simulink model "model_6dof"  (R2021b)
settings: Solver=ode4  StartTime=0  StopTime=stopt  FixedStep=ts  RelTol=1e-3
values from neighbouring files (symbols this model uses):
  d = 0.265    [totalfm.m]
  q = U(2)    [totalfm.m]
  r = U(3)    [totalfm.m]
  rail_len = U(4)    [stage_func.m]
undefined symbols (not defined in the file or in its folder): afa, alpha, atkinter, beta, caoff1000, caoff10000, caoff5000, caon1000, caon10000, caon5000, cl_phi1000, cl_phi10000, cl_phi5000, cldp1000, cldp10000, cldp5000, clp10000, clp5000, clpc_1000, clpt_1000, cma_1000, cmad_1000, cmdq10000, cmdq5000, cmq1000, cmq10000, cmq5000, cn1000, cn10000, cn5000, cna_1000, cndq1000, cnq1000, cnq10000, cnq5000, damp, ex0, ey0, ez0, HDBK, K1, K2, K3, KP, MIL, Minter, p0, pitch_control_on, q0, r0, roll_control_on, Severe, SIM_CASE, tou, tou1, tou2, ts, turb_on, u0, v0 ... (+14)
libraries: simulink x15, simulink_extras x5, aerolibasang x2, dspmathops x1, aerolibatmos2 x1, aerolibconvert2 x1, aerolibwind2 x1, mspsensorlib x1, sensorinslib x1, sharedtransform x1, vrlib x1
settings Model: Creator=a0972  LastModifiedBy=310611102
settings DataIOCC: SaveFormat=StructureWithTime
settings OptimizationCC: BlockReduction=off  BufferReuse=off
settings DebuggingCC: AlgebraicLoopMsg=none  UnconnectedInputMsg=none  UnconnectedOutputMsg=none  UnconnectedLineMsg=none

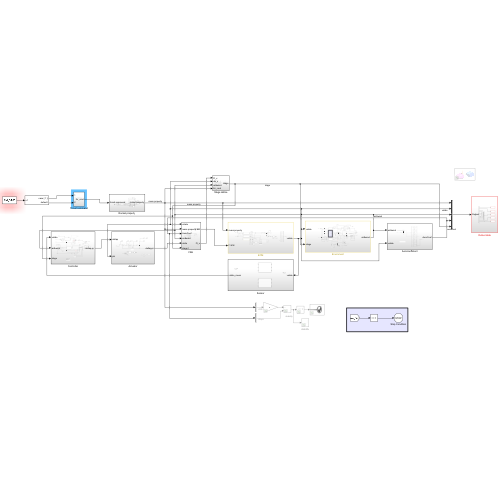
[thumbnail: Simulink's stored preview of the top-level diagram]
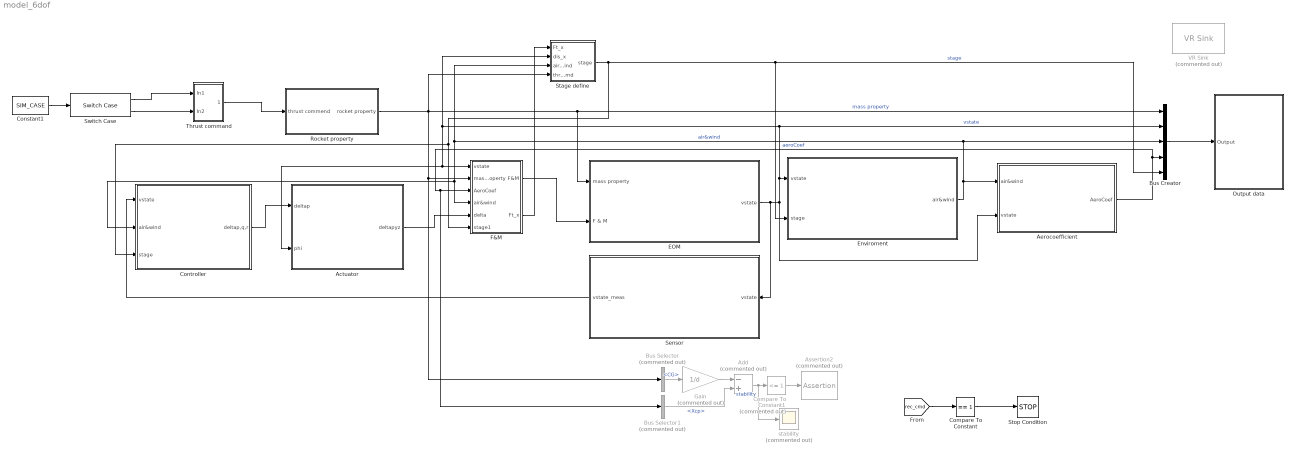
== system model_6dof ==
  Actuator : Subsystem
  Add : Sum  Commented=on  Inputs=-+
  Aerocoefficient : Subsystem
  Assertion2 : Assertion  Commented=on  AssertionFailFcn=error('unstable')
  Bus Creator : BusCreator  Inputs=5
  Bus Selector : BusSelector  Commented=on  OutputSignals=CG
  Bus Selector1 : BusSelector  Commented=on  OutputSignals=Xcp
  Compare To Constant : simulink/Logic and Bit Operations/Compare To Constant  relop===  const=1  OutDataTypeStr=boolean
  Compare To Constant1 : simulink/Logic and Bit Operations/Compare To Constant  Commented=on  relop=<=  const=1  OutDataTypeStr=boolean
  Constant1 : Constant  Value=SIM_CASE
  Controller : Subsystem
  EOM : Subsystem
  Enviroment : Subsystem
  F&M : Subsystem
  Gain : Gain  Commented=on  Gain=1/d
  Output data : Subsystem
  Rocket property : Subsystem
  Sensor : Subsystem
  Stage define : Subsystem
  Stop Condition : Stop
  Switch Case : SwitchCase
  Thrust command : Subsystem
  VR Sink : vrlib/VR Sink  Commented=on  InstantiateOnLoad=on  SampleTime=ts  ViewEnable=on  RemoteChange=off  RemoteView=off  AutoView=off  VideoDimensions=[]  AllowVariableSize=off
  stability : Scope  Commented=on
  wires:
  Controller/1(deltap,q,r) -> Actuator/1(deltap)
  Bus Creator/1 -> Output data/1(Output)
  EOM/1(vstate) -> Sensor/1(vstate), Bus Creator/2, F&M/1(vstate), Actuator/2(phi), Stage define/2(dis_x), Enviroment/1(vstate), Aerocoefficient/2(vstate)  "vstate"
  Rocket property/1(rocket property) -> Bus Selector/1, F&M/2(mass property), Stage define/4(thr_cmd), EOM/1(mass property), Bus Creator/1  "mass property"
  Aerocoefficient/1(AeroCoef) -> Bus Creator/4, Bus Selector1/1, F&M/3(AeroCoef)  "aeroCoef"
  Enviroment/1(air&wind) -> Stage define/3(air&wind), F&M/4(air&wind), Controller/2(air&wind), Bus Creator/3, Aerocoefficient/1(air&wind)  "air&wind"
  [rec_cmd] -> Compare To Constant/1
  F&M/1(F&M) -> EOM/2(F & M)
  Stage define/1(stage) -> Controller/3(stage), F&M/6(stage1), Bus Creator/5, Enviroment/2(stage)  "stage"
  F&M/2(Ft_x) -> Stage define/1(Ft_x)
  Compare To Constant/1 -> Stop Condition/1
  Bus Selector/1 -> Gain/1  "<CG>"
  Bus Selector1/1 -> Add/2  "<Xcp>"
  Gain/1 -> Add/1
  Add/1 -> stability/1, Compare To Constant1/1  "stability"
  Compare To Constant1/1 -> Assertion2/1
  Actuator/1(deltapyz) -> F&M/5(delta)
  Constant1/1 -> Switch Case/1
  Thrust command/1(thr_cmd) -> Rocket property/1(thrust commend)
  Switch Case/1 -> Thrust command/1(In1)
  Switch Case/2 -> Thrust command/2(In2)
  Sensor/1(vstate_meas) -> Controller/1(vstate)

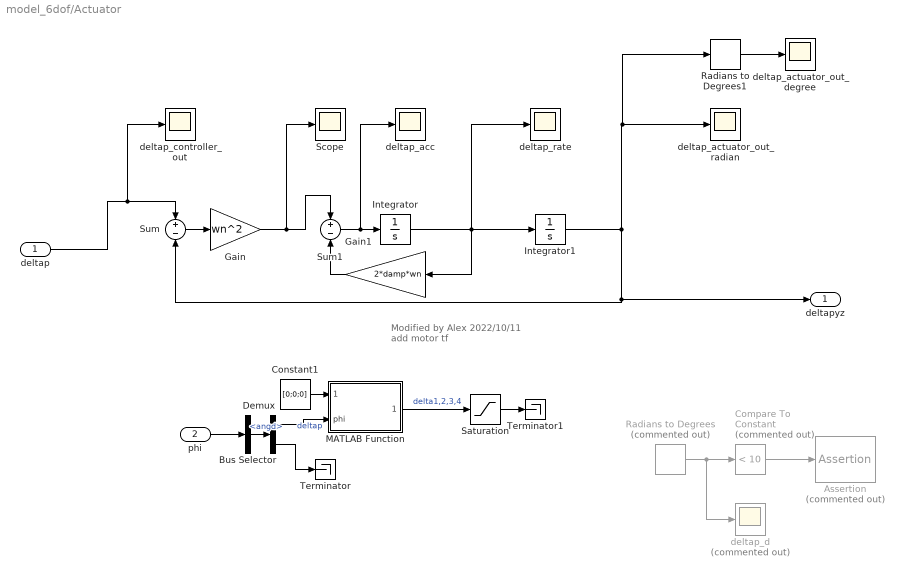
== system model_6dof/Actuator ==
  note: Modified by Alex
      | 2022/10/11
      | add motor tf
  deltap : Inport
  phi : Inport  Port=2
  Assertion : Assertion  Commented=on  AssertionFailFcn="error(\"large deflection angle\")"  StopWhenAssertionFail=off
  Bus Selector : BusSelector  OutputSignals=angd
  Compare To Constant : simulink/Logic and Bit Operations/Compare To Constant  Commented=on  relop=<  const=10  OutDataTypeStr=boolean
  Constant1 : Constant  Value=[0;0;0]
  Demux : Demux  Outputs=[1;2]
  Gain : Gain  Gain=wn^2
  Gain1 : Gain  Gain=2*damp*wn
  Integrator : Integrator
  Integrator1 : Integrator
  MATLAB Function : MATLAB Function  TreatAsAtomicUnit=on
  Radians to Degrees : simulink_extras/Transformations/Radians to Degrees  Commented=on
  Radians to Degrees1 : simulink_extras/Transformations/Radians to Degrees
  Saturation : Saturate
  Scope : Scope
  Sum : Sum  Inputs=+-
  Sum1 : Sum  Inputs=+-
  Terminator : Terminator
  Terminator1 : Terminator
  deltap_acc : Scope
  deltap_actuator_out_degree : Scope
  deltap_actuator_out_radian : Scope
  deltap_controller_out : Scope
  deltap_d : Scope  Commented=on
  deltap_rate : Scope
  deltapyz : Outport
  wires:
  MATLAB Function/1(delta1234) -> Saturation/1  "delta1,2,3,4"
  phi/1 -> Bus Selector/1
  Bus Selector/1 -> Demux/1  "<angd>"
  Demux/2 -> Terminator/1
  Integrator1/1 -> Sum/2, deltapyz/1, Radians to Degrees1/1, deltap_actuator_out_radian/1
  Saturation/1 -> Terminator1/1
  Constant1/1 -> MATLAB Function/1(deltapyz)
  Compare To Constant/1 -> Assertion/1
  Demux/1 -> MATLAB Function/2(phi)  "deltap"
  Radians to Degrees/1 -> deltap_d/1, Compare To Constant/1
  Sum/1 -> Gain/1
  Integrator/1 -> deltap_rate/1, Integrator1/1, Gain1/1
  Gain/1 -> Sum1/1, Scope/1
  Sum1/1 -> deltap_acc/1, Integrator/1
  deltap/1 -> deltap_controller_out/1, Sum/1
  Gain1/1 -> Sum1/2
  Radians to Degrees1/1 -> deltap_actuator_out_degree/1

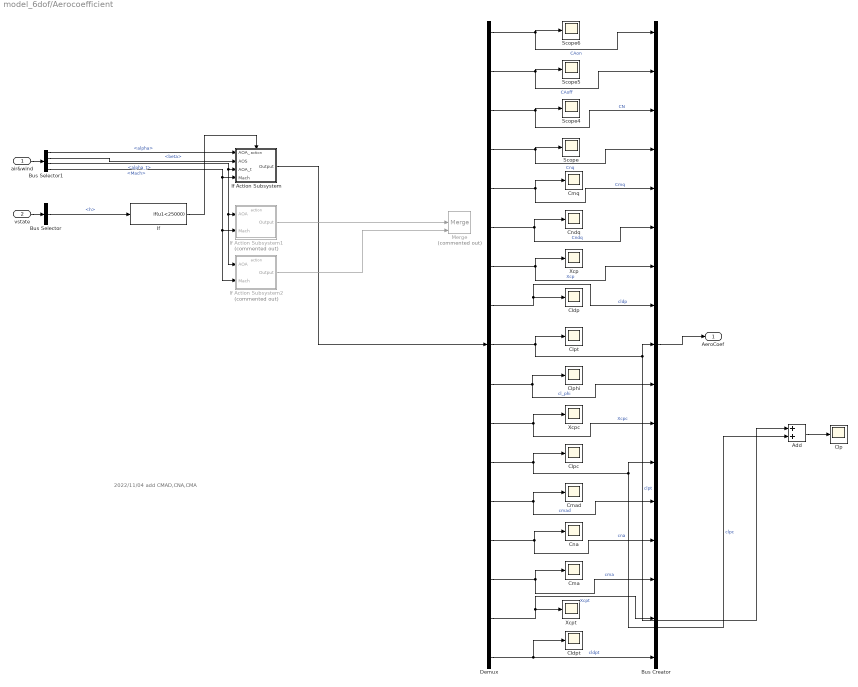
== system model_6dof/Aerocoefficient ==
  note: 2022/11/04 add CMAD,CNA,CMA
  air&wind : Inport
  vstate : Inport  Port=2
  Add : Sum
  Bus Creator : BusCreator  Inputs=17
  Bus Selector : BusSelector  OutputSignals=h
  Bus Selector1 : BusSelector  OutputSignals=AOA.alpha,AOA.beta,AOA.alpha_t,air.Mach
  Cldp : Scope
  Cldpt : Scope
  Clp : Scope
  Clpc : Scope
  Clphi : Scope
  Clpt : Scope
  Cma : Scope
  Cmad : Scope
  Cmq : Scope
  Cna : Scope
  Cndq : Scope
  Demux : Demux  Outputs=17
  If : If  IfExpression=u1<25000  ShowElse=off
  If Action Subsystem : Subsystem  TreatAsAtomicUnit=on
  If Action Subsystem1 : Subsystem  Commented=on  TreatAsAtomicUnit=on
  If Action Subsystem2 : Subsystem  Commented=on  TreatAsAtomicUnit=on
  Merge : Merge  Commented=on  Inputs=3
  Scope{,4..6} (4 alike) : Scope
  Xcp : Scope
  Xcpc : Scope
  Xcpt : Scope
  AeroCoef : Outport
  wires:
  If/1 -> If Action Subsystem/Action
  Demux/4 -> Bus Creator/4, Scope/1  "Cnq"
  Demux/1 -> Bus Creator/1, Scope6/1  "CAon"
  Demux/2 -> Bus Creator/2, Scope5/1  "CAoff"
  Demux/6 -> Bus Creator/6, Cndq/1  "Cndq"
  Demux/5 -> Bus Creator/5, Cmq/1  "Cmq"
  Demux/3 -> Bus Creator/3, Scope4/1  "CN"
  Demux/7 -> Xcp/1, Bus Creator/7  "Xcp"
  If Action Subsystem/1(Output) -> Demux/1
  If Action Subsystem1/1(Output) -> Merge/2
  If Action Subsystem2/1(Output) -> Merge/3
  Bus Selector1/3 -> If Action Subsystem2/1(AOA), If Action Subsystem1/1(AOA), If Action Subsystem/3(AOA_t)  "<alpha_t>"
  Bus Selector1/4 -> If Action Subsystem2/2(Mach), If Action Subsystem1/2(Mach), If Action Subsystem/4(Mach)  "<Mach>"
  Bus Creator/1 -> AeroCoef/1
  air&wind/1 -> Bus Selector1/1
  vstate/1 -> Bus Selector/1
  Bus Selector/1 -> If/1  "<h>"
  Demux/8 -> Bus Creator/8, Cldp/1  "cldp"
  Demux/9 -> Clpt/1, Add/1, Bus Creator/9  "clpt"
  Demux/10 -> Clphi/1, Bus Creator/10  "cl_phi"
  Demux/11 -> Xcpc/1, Bus Creator/11  "Xcpc"
  Demux/12 -> Clpc/1, Add/2, Bus Creator/12  "clpc"
  Bus Selector1/1 -> If Action Subsystem/1(AOA_)  "<alpha>"
  Bus Selector1/2 -> If Action Subsystem/2(AOS)  "<beta>"
  Add/1 -> Clp/1
  Demux/13 -> Cmad/1, Bus Creator/13  "cmad"
  Demux/14 -> Cna/1, Bus Creator/14  "cna"
  Demux/15 -> Cma/1, Bus Creator/15  "cma"
  Demux/16 -> Bus Creator/16, Xcpt/1  "Xcpt"
  Demux/17 -> Cldpt/1, Bus Creator/17  "cldpt"

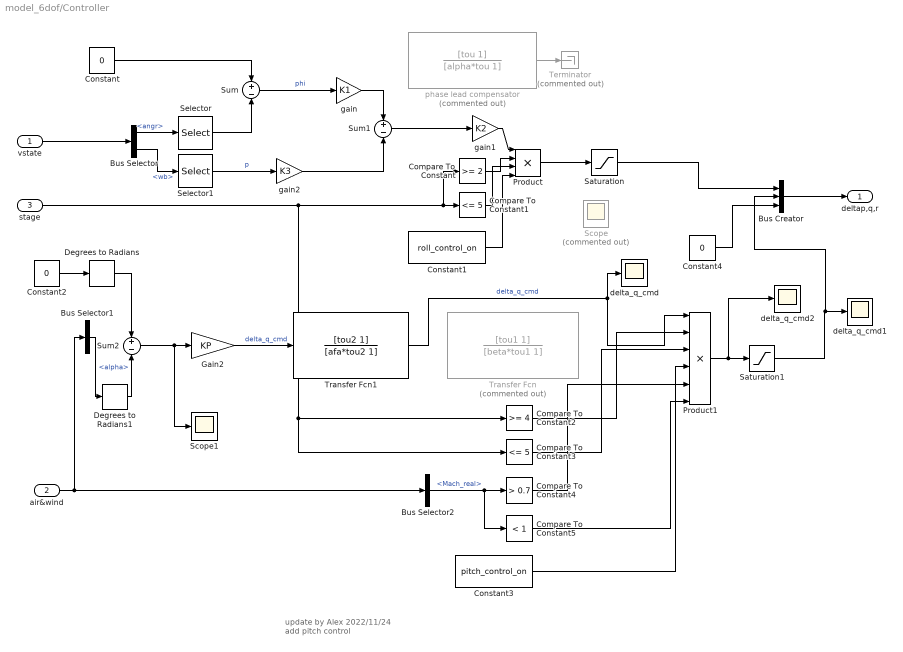
== system model_6dof/Controller ==
  note: update by Alex
      | 2022/11/24
      | add pitch control
  vstate : Inport
  air&wind : Inport  Port=2
  stage : Inport  Port=3
  Bus Creator : BusCreator  Inputs=3
  Bus Selector : BusSelector  OutputSignals=angr,wb
  Bus Selector1 : BusSelector  OutputSignals=AOA.alpha
  Bus Selector2 : BusSelector  OutputSignals=air.Mach_real
  Compare To Constant : simulink/Logic and Bit Operations/Compare To Constant  relop=>=  const=2  OutDataTypeStr=boolean
  Compare To Constant1 : simulink/Logic and Bit Operations/Compare To Constant  relop=<=  const=5  OutDataTypeStr=boolean
  Compare To Constant2 : simulink/Logic and Bit Operations/Compare To Constant  relop=>=  const=4  OutDataTypeStr=boolean
  Compare To Constant3 : simulink/Logic and Bit Operations/Compare To Constant  relop=<=  const=5  OutDataTypeStr=boolean
  Compare To Constant4 : simulink/Logic and Bit Operations/Compare To Constant  relop=>  const=0.7  OutDataTypeStr=boolean
  Compare To Constant5 : simulink/Logic and Bit Operations/Compare To Constant  relop=<  const=1  OutDataTypeStr=boolean
  Constant : Constant  Value=0
  Constant1 : Constant  Value=roll_control_on
  Constant2 : Constant  Value=0
  Constant3 : Constant  Value=pitch_control_on
  Constant4 : Constant  Value=0
  Degrees to Radians : simulink_extras/Transformations/Degrees to Radians
  Degrees to Radians1 : simulink_extras/Transformations/Degrees to Radians
  Gain2 : Gain  Gain=KP
  Product : Product  Inputs=4
  Product1 : Product  Inputs=6
  Saturation : Saturate  UpperLimit=10*pi/180  LowerLimit=-10*pi/180
  Saturation1 : Saturate  UpperLimit=10*pi/180  LowerLimit=-10*pi/180
  Scope : Scope  Commented=on
  Scope1 : Scope
  Selector : Selector  InputPortWidth=3  IndexOptions=Index vector (dialog)  Indices=[1]  OutputSizes=1
  Selector1 : Selector  InputPortWidth=3  IndexOptions=Index vector (dialog)  Indices=[1]  OutputSizes=1
  Sum : Sum  Inputs=+-
  Sum1 : Sum  Inputs=+-
  Sum2 : Sum  Inputs=+-
  Terminator : Terminator  Commented=on
  Transfer Fcn : TransferFcn  Commented=on  Numerator=[tou1 1]  Denominator=[beta*tou1 1]
  Transfer Fcn1 : TransferFcn  Numerator=[tou2 1]  Denominator=[afa*tou2 1]
  delta_q_cmd : Scope
  delta_q_cmd1 : Scope
  delta_q_cmd2 : Scope
  gain : Gain  Gain=K1
  gain1 : Gain  Gain=K2
  gain2 : Gain  Gain=K3
  phase lead compensator : TransferFcn  Commented=on  Numerator=[tou 1]  Denominator=[alpha*tou 1]
  deltap,q,r : Outport
  wires:
  gain/1 -> Sum1/1
  Constant/1 -> Sum/1
  vstate/1 -> Bus Selector/1
  Sum/1 -> gain/1  "phi"
  phase lead compensator/1 -> Terminator/1
  Bus Selector/1 -> Selector/1  "<angr>"
  Selector/1 -> Sum/2
  Bus Selector/2 -> Selector1/1  "<wb>"
  Selector1/1 -> gain2/1  "p"
  Sum1/1 -> gain1/1
  gain1/1 -> Product/1
  Compare To Constant/1 -> Product/2
  Compare To Constant1/1 -> Product/3
  Product/1 -> Saturation/1
  Constant1/1 -> Product/4
  Saturation/1 -> Bus Creator/1
  gain2/1 -> Sum1/2
  Constant2/1 -> Degrees to Radians/1
  air&wind/1 -> Bus Selector1/1, Bus Selector2/1
  Sum2/1 -> Scope1/1, Gain2/1
  Transfer Fcn1/1 -> Product1/1, delta_q_cmd/1  "delta_q_cmd"
  stage/1 -> Compare To Constant2/1, Compare To Constant3/1, Compare To Constant/1, Compare To Constant1/1
  Constant3/1 -> Product1/4
  Compare To Constant3/1 -> Product1/3
  Compare To Constant2/1 -> Product1/2
  Bus Selector2/1 -> Compare To Constant5/1, Compare To Constant4/1  "<Mach_real>"
  Compare To Constant5/1 -> Product1/6
  Compare To Constant4/1 -> Product1/5
  Constant4/1 -> Bus Creator/3
  Bus Creator/1 -> deltap,q,r/1
  Degrees to Radians/1 -> Sum2/1
  Bus Selector1/1 -> Degrees to Radians1/1  "<alpha>"
  Product1/1 -> Saturation1/1, delta_q_cmd2/1
  Saturation1/1 -> Bus Creator/2, delta_q_cmd1/1
  Gain2/1 -> Transfer Fcn1/1  "delta_q_cmd"
  Degrees to Radians1/1 -> Sum2/2

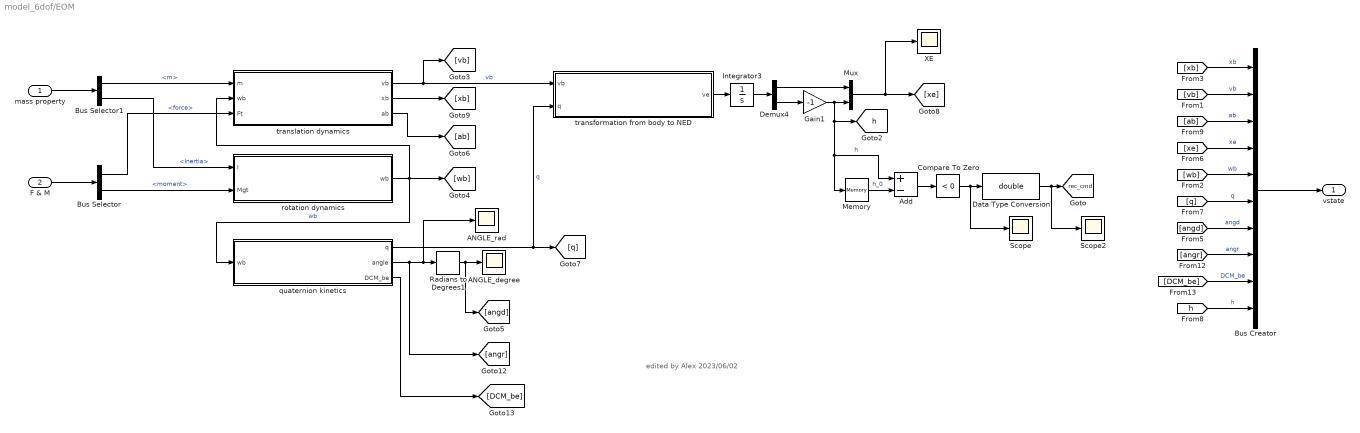
== system model_6dof/EOM ==
  note: edited by Alex
      | 2023/06/02
  mass property : Inport
  F & M : Inport  Port=2
  ANGLE_degree : Scope
  ANGLE_rad : Scope
  Add : Sum  Inputs=+-
  Bus Creator : BusCreator  Inputs=10
  Bus Selector : BusSelector  OutputSignals=force,moment
  Bus Selector1 : BusSelector  OutputSignals=m,Inertia
  Compare To Zero : simulink/Logic and Bit Operations/Compare To Zero  relop=<  OutDataTypeStr=boolean
  Data Type Conversion : DataTypeConversion  OutDataTypeStr=double
  Demux4 : Demux  Outputs=[2 1]
  Gain1 : Gain  Gain=-1
  Integrator3 : Integrator  InitialCondition=[x0;y0;z0]
  Memory : Memory
  Mux : Mux  Inputs=2
  Radians to Degrees1 : simulink_extras/Transformations/Radians to Degrees
  Scope : Scope
  Scope2 : Scope
  XE : Scope
  quaternion kinetics : Subsystem
  rotation dynamics : Subsystem
  transformation from body to NED : Subsystem
  translation dynamics : Subsystem
  vstate : Outport
  tag scope: h=global, rec_cmd=global
  wires:
  F & M/1 -> Bus Selector/1
  Bus Selector/1 -> translation dynamics/3(Ft)  "<force>"
  Bus Selector/2 -> rotation dynamics/2(Mgt)  "<moment>"
  rotation dynamics/1(wb) -> translation dynamics/2(wb), quaternion kinetics/1(wb), [wb]  "wb"
  Radians to Degrees1/1 -> ANGLE_degree/1, [angd]
  quaternion kinetics/2(angle) -> ANGLE_rad/1, Radians to Degrees1/1, [angr]
  translation dynamics/1(vb) -> [vb], transformation from body to NED/1(vb)  "vb"
  quaternion kinetics/1(q) -> transformation from body to NED/2(q), [q]  "q"
  Bus Creator/1 -> vstate/1
  Bus Selector1/1 -> translation dynamics/1(m)  "<m>"
  Bus Selector1/2 -> rotation dynamics/1(I)  "<Inertia>"
  mass property/1 -> Bus Selector1/1
  Demux4/1 -> Mux/1
  Gain1/1 -> Add/1, Memory/1, [h], Mux/2  "h"
  Demux4/2 -> Gain1/1
  transformation from body to NED/1(ve) -> Integrator3/1
  Integrator3/1 -> Demux4/1
  Mux/1 -> XE/1, [xe]
  translation dynamics/2(xb) -> [xb]
  [angd] -> Bus Creator/7  "angd"
  [xe] -> Bus Creator/4  "xe"
  [q] -> Bus Creator/6  "q"
  [h] -> Bus Creator/10  "h"
  [xb] -> Bus Creator/1  "xb"
  [vb] -> Bus Creator/2  "vb"
  translation dynamics/3(ab) -> [ab]
  [ab] -> Bus Creator/3  "ab"
  [wb] -> Bus Creator/5  "wb"
  [angr] -> Bus Creator/8  "angr"
  quaternion kinetics/3(DCM_be) -> [DCM_be]
  [DCM_be] -> Bus Creator/9  "DCM_be"
  Memory/1 -> Add/2  "h_0"
  Add/1 -> Compare To Zero/1
  Compare To Zero/1 -> Data Type Conversion/1, Scope/1
  Data Type Conversion/1 -> Scope2/1, [rec_cmd]

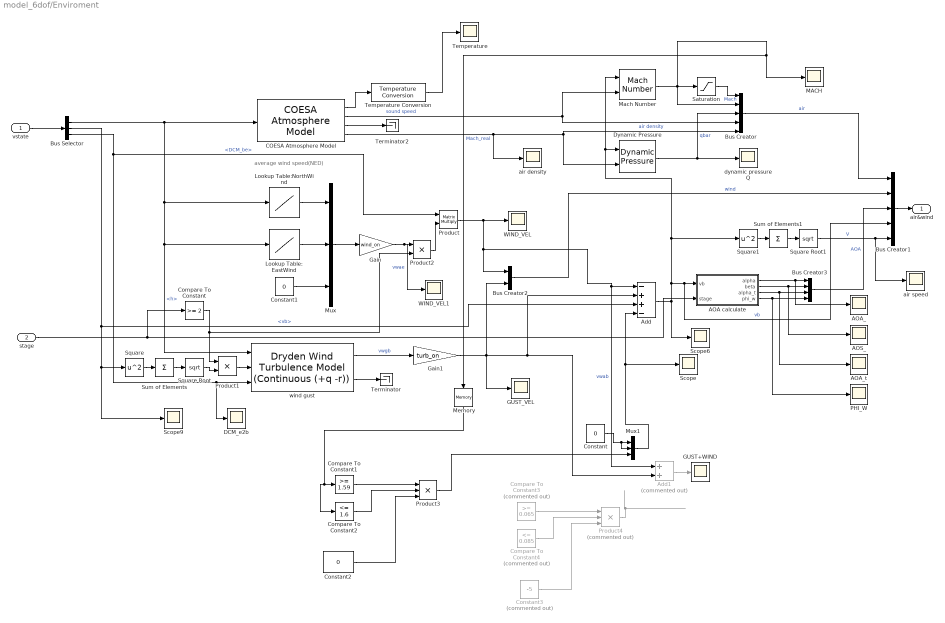
== system model_6dof/Enviroment ==
  note: average wind speed(NED)
  vstate : Inport
  stage : Inport  Port=2
  AOA calculate : MATLAB Function  TreatAsAtomicUnit=on
  AOA_ : Scope
  AOA_t : Scope
  AOS_ : Scope
  Add : Sum  Inputs=-++-
  Add1 : Sum  Commented=on
  Bus Creator : BusCreator  Inputs=5
  Bus Creator1 : BusCreator  Inputs=5
  Bus Creator2 : BusCreator  Inputs=2
  Bus Creator3 : BusCreator  Inputs=4
  Bus Selector : BusSelector  OutputSignals=h,vb,DCM_be
  COESA Atmosphere Model : aerolibatmos2/COESA Atmosphere Model  units=Metric (MKS)  spec=1976 COESA-extended U.S. Standard Atmosphere  model=Profile  profile_var=High temperature  profile_percent=1%  profile_alt=5 km (16404 ft)  envelope_var=High temperature  envelope_percent=1%  action=Warning
  Compare To Constant : simulink/Logic and Bit Operations/Compare To Constant  relop=>=  const=2  OutDataTypeStr=boolean
  Compare To Constant1 : simulink/Logic and Bit Operations/Compare To Constant  relop=>=  const=1.59  OutDataTypeStr=boolean
  Compare To Constant2 : simulink/Logic and Bit Operations/Compare To Constant  relop=<=  const=1.6  OutDataTypeStr=boolean
  Compare To Constant3 : simulink/Logic and Bit Operations/Compare To Constant  Commented=on  relop=>=  const=0.065  OutDataTypeStr=boolean
  Compare To Constant4 : simulink/Logic and Bit Operations/Compare To Constant  Commented=on  relop=<=  const=0.085  OutDataTypeStr=boolean
  Constant : Constant  Value=0
  Constant1 : Constant  Value=0
  Constant2 : Constant  Value=0
  Constant3 : Constant  Commented=on  Value=-5
  DCM_e2b : Scope
  Dynamic Pressure : aerolibasang/Dynamic Pressure
  GUST+WIND : Scope
  GUST_VEL : Scope
  Gain : Gain  Gain=wind_on
  Gain1 : Gain  Gain=turb_on
  Lookup Table: EastWind : Lookup  InputValues=wind_h  Table=wind_east  LookUpMeth=Interpolation-Use End Values
  Lookup Table:NorthWind : Lookup  InputValues=wind_h  Table=wind_north  LookUpMeth=Interpolation-Use End Values
  MACH : Scope
  Mach Number : aerolibasang/Mach Number
      settings: SourceProductBaseCode=AE
  Memory : Memory
  Mux : Mux  Inputs=3
  Mux1 : Mux  Inputs=3
  PHI_W : Scope
  Product : Product  Multiplication=Matrix(*)
  Product1 : Product
  Product2 : Product
  Product3 : Product  Inputs=3
  Product4 : Product  Commented=on  Inputs=3
  Saturation : Saturate  UpperLimit=1.8  LowerLimit=0.1
  Scope : Scope
  Scope6 : Scope
  Scope9 : Scope
  Square : Math  Operator=square  SignedPower=on  SaturateOnIntegerOverflow=on
  Square Root : Sqrt  SaturateOnIntegerOverflow=on
  Square Root1 : Sqrt  SaturateOnIntegerOverflow=on
  Square1 : Math  Operator=square  SignedPower=on  SaturateOnIntegerOverflow=on
  Sum of Elements : Sum  Inputs=+
  Sum of Elements1 : Sum  Inputs=+
  Temperature : Scope
  Temperature Conversion : aerolibconvert2/Temperature Conversion  IU=K  OU=C
      settings: SourceProductBaseCode=AE
  Terminator : Terminator
  Terminator2 : Terminator
  WIND_VEL : Scope
  WIND_VEL1 : Scope
  air density : Scope
  air speed : Scope
  dynamic pressure Q : Scope
  wind gust : aerolibwind2/Dryden Wind Turbulence Model  (Continuous (+q -r))  units=Metric (MKS)  spec=MIL-HDBK-1797B  model=Discrete Dryden (+q -r)  W20=5  Wdeg=45  TurbProb=10^-5 - Severe  L_high=533.4  Wingspan=0.5  ts=ts  Seed=[23341 23342 23343 23344]  T_on=on
  air&wind : Outport
  wires:
  vstate/1 -> Bus Selector/1
  Bus Selector/1 -> wind gust/1, Lookup Table: EastWind/1, Lookup Table:NorthWind/1, COESA Atmosphere Model/1  "<h>"
  COESA Atmosphere Model/2 -> Mach Number/2, Bus Creator/4  "sound speed"
  COESA Atmosphere Model/4 -> air density/1, Bus Creator/5, Dynamic Pressure/2  "air density"
  Mux/1 -> Gain/1
  Sum of Elements/1 -> Square Root/1
  wind gust/2 -> Terminator/1
  Square/1 -> Sum of Elements/1
  Lookup Table:NorthWind/1 -> Mux/1
  Lookup Table: EastWind/1 -> Mux/2
  Bus Selector/2 -> Add/3, Scope9/1, Square/1  "<vb>"
  wind gust/1 -> Gain1/1  "vwgb"
  Constant1/1 -> Mux/3
  Bus Creator1/1 -> air&wind/1
  Bus Creator/1 -> Bus Creator1/1  "air"
  Bus Creator2/1 -> Bus Creator1/2  "wind"
  Bus Selector/3 -> DCM_e2b/1, wind gust/3, Product/1  "<DCM_be>"
  Gain/1 -> WIND_VEL1/1, Product2/1  "vwae"
  Product/1 -> WIND_VEL/1, Add1/1, Add/1, Bus Creator2/1  "vwab"
  COESA Atmosphere Model/1 -> Temperature Conversion/1
  COESA Atmosphere Model/3 -> Terminator2/1
  Mach Number/1 -> Bus Creator/2, Memory/1, MACH/1, Saturation/1  "Mach_real"
  Dynamic Pressure/1 -> Bus Creator/3, dynamic pressure Q/1  "qbar"
  Saturation/1 -> Bus Creator/1  "Mach"
  AOA calculate/1(alpha) -> Bus Creator3/1, AOA_/1
  AOA calculate/2(beta) -> Bus Creator3/2, AOS_/1
  AOA calculate/3(alpha_t) -> AOA_t/1, Bus Creator3/3
  AOA calculate/4(phi_w) -> PHI_W/1, Bus Creator3/4
  Bus Creator3/1 -> Bus Creator1/3  "AOA"
  stage/1 -> AOA calculate/2(stage), Compare To Constant/1
  Square Root1/1 -> air speed/1, Bus Creator1/5  "V"
  Sum of Elements1/1 -> Square Root1/1
  Add/1 -> Dynamic Pressure/1, Mach Number/1, Square1/1, Bus Creator1/4, AOA calculate/1(vb), Scope6/1  "vb"
  Square1/1 -> Sum of Elements1/1
  Compare To Constant/1 -> Product2/2, Product1/1
  Square Root/1 -> Product1/2
  Product1/1 -> wind gust/2
  Add1/1 -> GUST+WIND/1
  Gain1/1 -> GUST_VEL/1, Add1/2, Add/2, Bus Creator2/2
  Product2/1 -> Product/2
  Compare To Constant1/1 -> Product3/1
  Compare To Constant2/1 -> Product3/2
  Constant/1 -> Mux1/2, Mux1/1
  Constant2/1 -> Product3/3
  Mux1/1 -> Scope/1, Add/4
  Memory/1 -> Compare To Constant2/1, Compare To Constant1/1
  Compare To Constant4/1 -> Product4/2
  Product4/1 -> ?
  Compare To Constant3/1 -> Product4/1
  Constant3/1 -> Product4/3
  ? -> Compare To Constant4/1, Compare To Constant3/1
  Product3/1 -> Mux1/3
  Temperature Conversion/1 -> Temperature/1

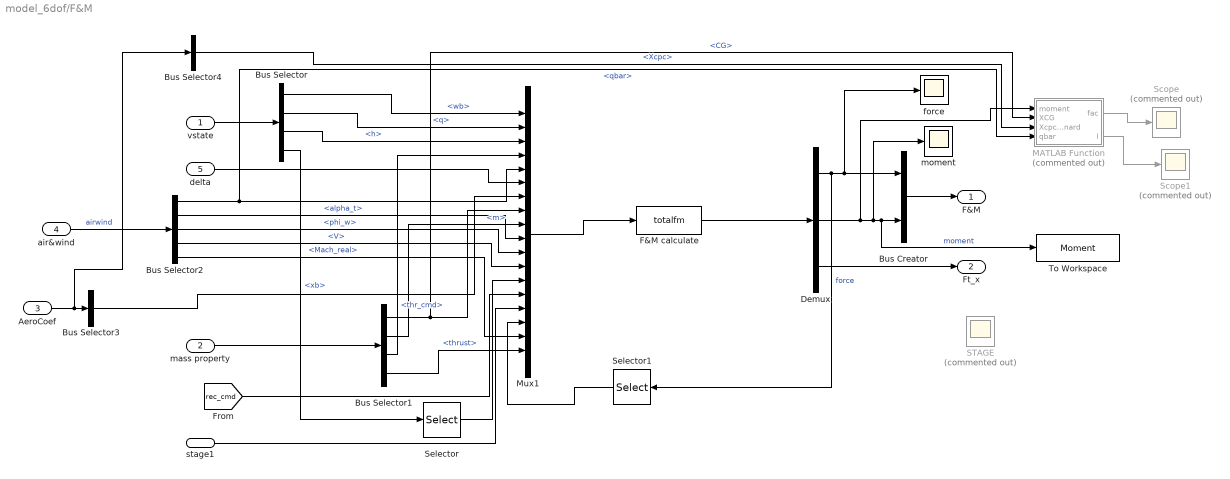
== system model_6dof/F&M ==
  vstate : Inport
  mass property : Inport  Port=2
  AeroCoef : Inport  Port=3
  air&wind : Inport  Port=4
  delta : Inport  Port=5
  stage1 : Inport  Port=6
  Bus Creator : BusCreator  Inputs=2
  Bus Selector : BusSelector  OutputSignals=wb,q,h,xb
  Bus Selector1 : BusSelector  OutputSignals=CG,m,thr_cmd,thrust
  Bus Selector2 : BusSelector  OutputSignals=air.qbar,AOA.alpha_t,AOA.phi_w,V,air.Mach_real
  Bus Selector3 : BusSelector  OutputSignals=CAon,CAoff,CN,Cnq,Cmq,Cndq,Xcp,cldp,clpt,cl_phi,Xcpc,clpc,cldpt  OutputAsBus=on
  Bus Selector4 : BusSelector  OutputSignals=Xcpc
  Demux : Demux  Outputs=[3 3 1]
  F&M calculate : MATLABFcn  MATLABFcn=totalfm  OutputDimensions=7
  MATLAB Function : MATLAB Function  Commented=on  TreatAsAtomicUnit=on
  Mux1 : Mux  Inputs=[3 4 1 1 1 3 13 1 1 1 1 1 1 1 1 1 1 1]
  STAGE : Scope  Commented=on
  Scope : Scope  Commented=on
  Scope1 : Scope  Commented=on
  Selector : Selector  InputPortWidth=3  IndexOptions=Index vector (dialog)  Indices=[1]  OutputSizes=1
  Selector1 : Selector  InputPortWidth=3  IndexOptions=Index vector (dialog)  Indices=[1]  OutputSizes=1
  To Workspace : ToWorkspace  VariableName=Moment  SampleTime=-1
  force : Scope
  moment : Scope
  F&M : Outport
  Ft_x : Outport  Port=2
  wires:
  Demux/2 -> MATLAB Function/1(moment), To Workspace/1, Bus Creator/2, moment/1  "moment"
  Demux/1 -> Selector1/1, force/1, Bus Creator/1  "force"
  F&M calculate/1 -> Demux/1
  delta/1 -> Mux1/6
  Bus Selector/3 -> Mux1/3  "<h>"
  Bus Selector1/1 -> MATLAB Function/2(XCG), Mux1/8  "<CG>"
  vstate/1 -> Bus Selector/1
  Bus Selector/1 -> Mux1/1  "<wb>"
  Bus Selector/2 -> Mux1/2  "<q>"
  mass property/1 -> Bus Selector1/1
  Bus Selector1/2 -> Mux1/9  "<m>"
  Bus Selector2/1 -> MATLAB Function/4(qbar), Mux1/5  "<qbar>"
  Bus Selector3/1 -> Mux1/7
  Mux1/1 -> F&M calculate/1
  air&wind/1 -> Bus Selector2/1  "airwind"
  Bus Selector1/3 -> Mux1/4  "<thr_cmd>"
  Bus Creator/1 -> F&M/1
  Demux/3 -> Ft_x/1
  Bus Selector2/2 -> Mux1/10  "<alpha_t>"
  Bus Selector2/3 -> Mux1/11  "<phi_w>"
  Bus Selector2/4 -> Mux1/12  "<V>"
  Bus Selector/4 -> Selector/1  "<xb>"
  Selector/1 -> Mux1/13
  [rec_cmd] -> Mux1/14
  Selector1/1 -> Mux1/16
  Bus Selector2/5 -> Mux1/17  "<Mach_real>"
  stage1/1 -> Mux1/15
  AeroCoef/1 -> Bus Selector4/1, Bus Selector3/1
  MATLAB Function/1(fac) -> Scope/1
  Bus Selector4/1 -> MATLAB Function/3(Xcpcanard)  "<Xcpc>"
  MATLAB Function/2(l) -> Scope1/1
  Bus Selector1/4 -> Mux1/18  "<thrust>"

== system model_6dof/Output data ==
  Output : Inport
  Bus Creator : BusCreator  Inputs=7
  Bus Selector : BusSelector  OutputSignals=mass property,aeroCoef,vstate.xb,vstate.vb,vstate.ab,vstate.xe,vstate.wb,vstate.q,vstate.angd,air&wind,stage
  To Workspace1 : ToWorkspace  VariableName=vstate  SampleTime=-1
  To Workspace12 : ToWorkspace  VariableName=aeroCoef  SampleTime=-1
  To Workspace13 : ToWorkspace  VariableName=air  SampleTime=-1
  To Workspace6 : ToWorkspace  VariableName=stage  SampleTime=-1
  To Workspace9 : ToWorkspace  VariableName=mass_property  SaveFormat=Structure With Time  SampleTime=-1
  wires:
  Output/1 -> Bus Selector/1
  Bus Selector/1 -> To Workspace9/1  "<mass property>"
  Bus Selector/2 -> To Workspace12/1  "<aeroCoef>"
  Bus Selector/10 -> To Workspace13/1  "<air&wind>"
  Bus Selector/11 -> To Workspace6/1  "<stage>"
  Bus Selector/9 -> Bus Creator/7  "<angd>"
  Bus Selector/8 -> Bus Creator/6  "<q>"
  Bus Selector/7 -> Bus Creator/5  "<wb>"
  Bus Selector/6 -> Bus Creator/4  "<xe>"
  Bus Selector/5 -> Bus Creator/3  "<ab>"
  Bus Selector/4 -> Bus Creator/2  "<vb>"
  Bus Selector/3 -> Bus Creator/1  "<xb>"
  Bus Creator/1 -> To Workspace1/1

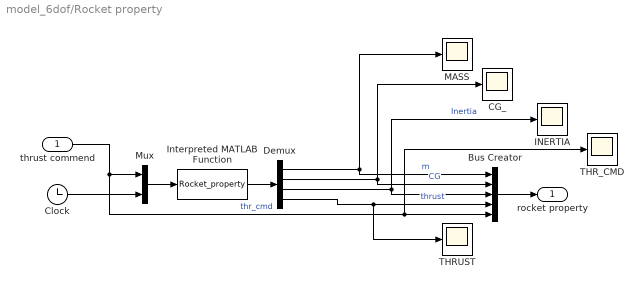
== system model_6dof/Rocket property ==
  thrust commend : Inport
  Bus Creator : BusCreator  Inputs=5
  CG_ : Scope
  Clock : Clock
  Demux : Demux  Outputs=[1 1 3 1]
  INERTIA : Scope
  Interpreted MATLAB Function : MATLABFcn  MATLABFcn=Rocket_property  OutputDimensions=6
  MASS : Scope
  Mux : Mux  Inputs=2
  THRUST : Scope
  THR_CMD : Scope
  rocket property : Outport
  wires:
  thrust commend/1 -> THR_CMD/1, Bus Creator/5, Mux/1  "thr_cmd"
  Clock/1 -> Mux/2
  Demux/3 -> Bus Creator/3, INERTIA/1  "Inertia"
  Demux/2 -> Bus Creator/2, CG_/1  "CG"
  Demux/1 -> MASS/1, Bus Creator/1  "m"
  Bus Creator/1 -> rocket property/1
  Interpreted MATLAB Function/1 -> Demux/1
  Mux/1 -> Interpreted MATLAB Function/1
  Demux/4 -> THRUST/1, Bus Creator/4  "thrust"

== system model_6dof/Sensor ==
  vstate : Inport
  Bus Selector : BusSelector  OutputSignals=signal1,signal2
  IMU : mspsensorlib/IMU  DispRefFrame=NED  Temperature=25  MagneticFieldNED=[ 27.5550, -2.4169, -16.0849 ]  MagneticFieldENU=[ -2.4169, 27.5550, 16.0849 ]  SeedDouble=67  SimulateUsing=Interpreted execution  AccelParamsMeasurementRange=Inf  AccelParamsResolution=0  AccelParamsConstantBias=[ 0, 0, 0 ]  AccelParamsAxesMisalignment=[ 100, 0, 0; 0, 100, 0; 0, 0, 100 ]  AccelParamsNoiseDensity=[ 0, 0, 0 ]  AccelParamsBiasInstability=[ 0, 0, 0 ]  AccelParamsRandomWalk=[ 0, 0, 0 ]  AccelParamsTemperatureBias=[ 0, 0, 0 ]  AccelParamsTemperatureScaleFactor=[ 0, 0, 0 ]  GyroParamsMeasurementRange=Inf  GyroParamsResolution=0  GyroParamsConstantBias=[ 0, 0, 0 ]  GyroParamsAxesMisalignment=[ 100, 0, 0; 0, 100, 0; 0, 0, 100 ]  GyroParamsAccelerationBias=[ 0, 0, 0 ]  GyroParamsNoiseDensity=[ 0, 0, 0 ]  GyroParamsBiasInstability=[ 0, 0, 0 ]  GyroParamsRandomWalk=[ 0, 0, 0 ]  GyroParamsTemperatureBias=[ 0, 0, 0 ]  GyroParamsTemperatureScaleFactor=[ 0, 0, 0 ]  MagParamsMeasurementRange=Inf  MagParamsResolution=0  MagParamsConstantBias=[ 0, 0, 0 ]  MagParamsAxesMisalignment=[ 100, 0, 0; 0, 100, 0; 0, 0, 100 ]  MagParamsNoiseDensity=[ 0, 0, 0 ]  MagParamsBiasInstability=[ 0, 0, 0 ]  MagParamsRandomWalk=[ 0, 0, 0 ]  MagParamsTemperatureBias=[ 0, 0, 0 ]  MagParamsTemperatureScaleFactor=[ 0, 0, 0 ]
      settings: SourceProductBaseCode=TF,NV
  INS : sensorinslib/INS  MountingLocation=[0 0 0]  RollAccuracy=0.2  PitchAccuracy=0.2  YawAccuracy=1  PositionAccuracy=1  VelocityAccuracy=0.05  UseAccelAndAngVel=off  AccelerationAccuracy=0  AngularVelocityAccuracy=0  TimeInput=off  PositionErrorFactor=[0 0 0]  SeedDouble=67  SimulateUsing=Code generation
      settings: SourceProductBaseCode=DR,TF,NV,UV
  Rotation Angles to Direction Cosine Matrix : sharedtransform/Rotation Angles to Direction Cosine Matrix  rotationOrder=ZYX  aMode=aMode
      settings: SourceProductBaseCode=AE,PW,DR,MT,UV,VE
  vstate_meas : Outport
  wires:
  Rotation Angles to Direction Cosine Matrix/1 -> IMU/3

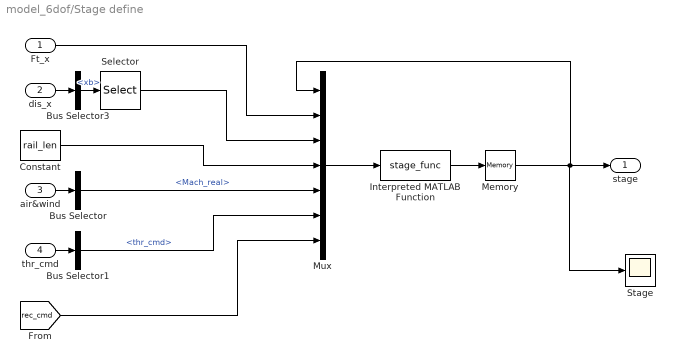
== system model_6dof/Stage define ==
  Ft_x : Inport
  dis_x : Inport  Port=2
  air&wind : Inport  Port=3
  thr_cmd : Inport  Port=4
  Bus Selector : BusSelector  OutputSignals=air.Mach_real
  Bus Selector1 : BusSelector  OutputSignals=thr_cmd
  Bus Selector3 : BusSelector  OutputSignals=xb
  Constant : Constant  Value=rail_len
  Interpreted MATLAB Function : MATLABFcn  MATLABFcn=stage_func  OutputDimensions=1
  Memory : Memory
  Mux : Mux  Inputs=7
  Selector : Selector  InputPortWidth=3  IndexOptions=Index vector (dialog)  Indices=[1]  OutputSizes=1
  Stage : Scope
  stage : Outport
  wires:
  Interpreted MATLAB Function/1 -> Memory/1
  Constant/1 -> Mux/4
  Memory/1 -> Stage/1, Mux/1, stage/1
  air&wind/1 -> Bus Selector/1
  Bus Selector/1 -> Mux/5  "<Mach_real>"
  thr_cmd/1 -> Bus Selector1/1
  Bus Selector1/1 -> Mux/6  "<thr_cmd>"
  [rec_cmd] -> Mux/7
  Ft_x/1 -> Mux/2
  Selector/1 -> Mux/3
  dis_x/1 -> Bus Selector3/1
  Bus Selector3/1 -> Selector/1  "<xb>"
  Mux/1 -> Interpreted MATLAB Function/1

== system model_6dof/Thrust command ==
  In1 : Inport
  In2 : Inport  Port=2
  Clock : Clock
  Constant : Constant
  thrust commend(0/1) : MATLAB Function  TreatAsAtomicUnit=on
  thr_cmd : Outport
  wires:
  thrust commend(0/1)/1(thr_cmd) -> thr_cmd/1
  Clock/1 -> thrust commend(0/1)/2(t)
  Constant/1 -> thrust commend(0/1)/1(thr)

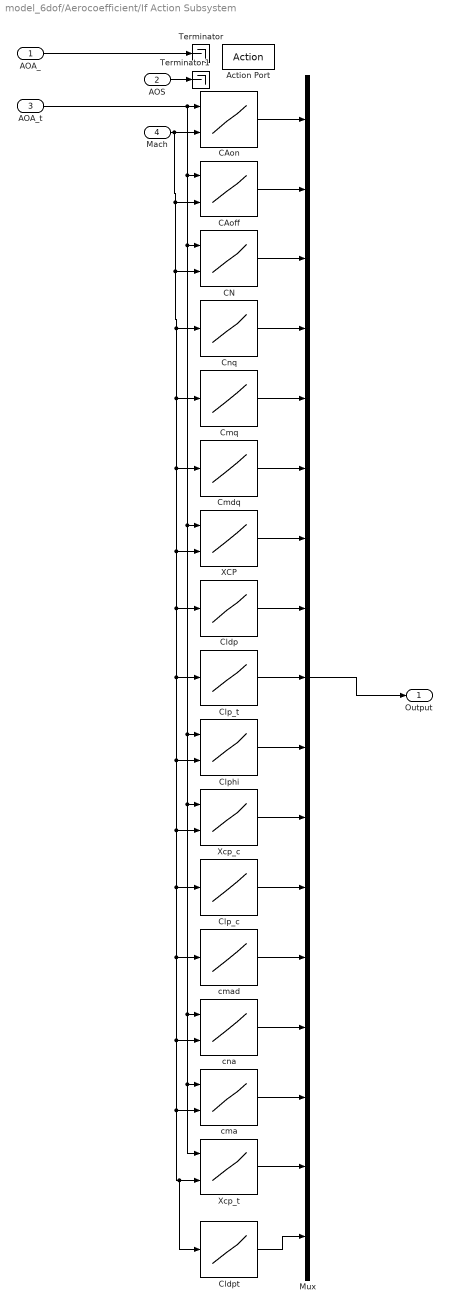
== system model_6dof/Aerocoefficient/If Action Subsystem ==
  AOA_ : Inport
  AOS : Inport  Port=2
  AOA_t : Inport  Port=3
  Mach : Inport  Port=4
  Action Port : ActionPort  ActionPortLabel=if(u1<25000)
  CAoff : Lookup_n-D  BreakpointsForDimension1=atkinter  BreakpointsForDimension2=Minter  Table=caoff1000  InternalRulePriority=Speed  RndMeth=Simplest  InputSameDT=on
      settings: InputPortMap=u0,u1
  CAon : Lookup_n-D  BreakpointsForDimension1=atkinter  BreakpointsForDimension2=Minter  Table=caon1000  InternalRulePriority=Speed  RndMeth=Simplest  InputSameDT=on
      settings: InputPortMap=u0,u1
  CN : Lookup_n-D  BreakpointsForDimension1=atkinter  BreakpointsForDimension2=Minter  Table=cn1000  InternalRulePriority=Speed  RndMeth=Simplest  InputSameDT=on
      settings: InputPortMap=u0,u1
  Cldp : Lookup_n-D  NumberOfTableDimensions=1  BreakpointsForDimension1=Minter  Table=cldp1000  InternalRulePriority=Speed  RndMeth=Simplest  InputSameDT=on
  Cldpt : Lookup_n-D  NumberOfTableDimensions=1  BreakpointsForDimension1=Minter  Table=cldp1000  InternalRulePriority=Speed  RndMeth=Simplest  InputSameDT=on
  Clp_c : Lookup_n-D  NumberOfTableDimensions=1  BreakpointsForDimension1=Minter  Table=clpc_1000  InternalRulePriority=Speed  RndMeth=Simplest  InputSameDT=on
  Clp_t : Lookup_n-D  NumberOfTableDimensions=1  BreakpointsForDimension1=Minter  Table=clpt_1000  InternalRulePriority=Speed  RndMeth=Simplest  InputSameDT=on
  Clphi : Lookup_n-D  BreakpointsForDimension1=atkinter  BreakpointsForDimension2=Minter  Table=cl_phi1000  InternalRulePriority=Speed  RndMeth=Simplest  InputSameDT=on
      settings: InputPortMap=u0,u1
  Cmdq : Lookup_n-D  NumberOfTableDimensions=1  BreakpointsForDimension1=Minter  Table=cndq1000  InternalRulePriority=Speed  RndMeth=Simplest  InputSameDT=on
  Cmq : Lookup_n-D  NumberOfTableDimensions=1  BreakpointsForDimension1=Minter  Table=cmq1000  InternalRulePriority=Speed  RndMeth=Simplest  InputSameDT=on
  Cnq : Lookup_n-D  NumberOfTableDimensions=1  BreakpointsForDimension1=Minter  Table=cnq1000  InternalRulePriority=Speed  RndMeth=Simplest  InputSameDT=on
  Mux : Mux  Inputs=17
  Terminator : Terminator
  Terminator1 : Terminator
  XCP : Lookup_n-D  BreakpointsForDimension1=atkinter  BreakpointsForDimension2=Minter  Table=xcp1000  InternalRulePriority=Speed  RndMeth=Simplest  InputSameDT=on
      settings: InputPortMap=u0,u1
  Xcp_c : Lookup_n-D  BreakpointsForDimension1=atkinter  BreakpointsForDimension2=Minter  Table=xcp_c1000  InternalRulePriority=Speed  RndMeth=Simplest  InputSameDT=on
      settings: InputPortMap=u0,u1
  Xcp_t : Lookup_n-D  BreakpointsForDimension1=atkinter  BreakpointsForDimension2=Minter  Table=xcp_t1000  InternalRulePriority=Speed  RndMeth=Simplest  InputSameDT=on
      settings: InputPortMap=u0,u1
  cma : Lookup_n-D  BreakpointsForDimension1=atkinter  BreakpointsForDimension2=Minter  Table=cma_1000  InternalRulePriority=Speed  RndMeth=Simplest  InputSameDT=on
      settings: InputPortMap=u0,u1
  cmad : Lookup_n-D  NumberOfTableDimensions=1  BreakpointsForDimension1=Minter  Table=cmad_1000  InternalRulePriority=Speed  RndMeth=Simplest  InputSameDT=on
  cna : Lookup_n-D  BreakpointsForDimension1=atkinter  BreakpointsForDimension2=Minter  Table=cna_1000  InternalRulePriority=Speed  RndMeth=Simplest  InputSameDT=on
      settings: InputPortMap=u0,u1
  Output : Outport
  wires:
  Cmq/1 -> Mux/5
  XCP/1 -> Mux/7
  CAoff/1 -> Mux/2
  Cmdq/1 -> Mux/6
  Cnq/1 -> Mux/4
  CN/1 -> Mux/3
  CAon/1 -> Mux/1
  Mux/1 -> Output/1
  Cldp/1 -> Mux/8
  Clp_t/1 -> Mux/9
  Clphi/1 -> Mux/10
  Xcp_c/1 -> Mux/11
  Clp_c/1 -> Mux/12
  AOA_/1 -> Terminator/1
  AOS/1 -> Terminator1/1
  AOA_t/1 -> CN/1, Xcp_t/1, cma/1, cna/1, Xcp_c/1, Clphi/1, XCP/1, CAoff/1, CAon/1
  cmad/1 -> Mux/13
  cna/1 -> Mux/14
  cma/1 -> Mux/15
  Xcp_t/1 -> Mux/16
  Mach/1 -> CN/2, Cldpt/1, Xcp_t/2, cma/2, cna/2, cmad/1, Clp_c/1, Xcp_c/2, Clphi/2, Clp_t/1, Cldp/1, XCP/2, Cmdq/1, Cmq/1, Cnq/1, CAoff/2, CAon/2
  Cldpt/1 -> Mux/17

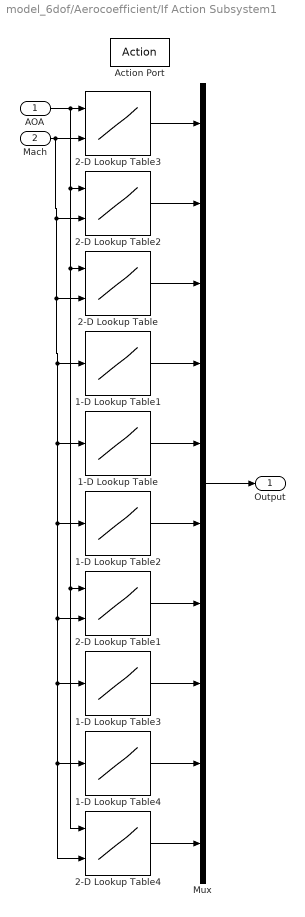
== system model_6dof/Aerocoefficient/If Action Subsystem1 ==
  AOA : Inport
  Mach : Inport  Port=2
  Action Port : ActionPort  ActionPortLabel=elseif(u1<10000)
  1-D Lookup Table : Lookup_n-D  NumberOfTableDimensions=1  BreakpointsForDimension1=Minter  Table=cmq5000  InterpMethod=Cubic spline  ExtrapMethod=Clip  InternalRulePriority=Speed  RndMeth=Simplest  InputSameDT=on
  1-D Lookup Table1 : Lookup_n-D  NumberOfTableDimensions=1  BreakpointsForDimension1=Minter  Table=cnq5000  InterpMethod=Cubic spline  ExtrapMethod=Clip  InternalRulePriority=Speed  RndMeth=Simplest  InputSameDT=on
  1-D Lookup Table2 : Lookup_n-D  NumberOfTableDimensions=1  BreakpointsForDimension1=Minter  Table=cmdq5000  InterpMethod=Cubic spline  ExtrapMethod=Clip  InternalRulePriority=Speed  RndMeth=Simplest  InputSameDT=on
  1-D Lookup Table3 : Lookup_n-D  NumberOfTableDimensions=1  BreakpointsForDimension1=Minter  Table=cldp5000  InterpMethod=Cubic spline  ExtrapMethod=Clip  InternalRulePriority=Speed  RndMeth=Simplest  InputSameDT=on
  1-D Lookup Table4 : Lookup_n-D  NumberOfTableDimensions=1  BreakpointsForDimension1=Minter  Table=clp5000  InterpMethod=Cubic spline  ExtrapMethod=Clip  InternalRulePriority=Speed  RndMeth=Simplest  InputSameDT=on
  2-D Lookup Table : Lookup_n-D  BreakpointsForDimension1=atkinter  BreakpointsForDimension2=Minter  Table=cn5000  InterpMethod=Cubic spline  ExtrapMethod=Clip  InternalRulePriority=Speed  RndMeth=Simplest  InputSameDT=on
      settings: InputPortMap=u0,u1
  2-D Lookup Table1 : Lookup_n-D  BreakpointsForDimension1=atkinter  BreakpointsForDimension2=Minter  Table=Xcp5000  InterpMethod=Cubic spline  ExtrapMethod=Clip  InternalRulePriority=Speed  RndMeth=Simplest  InputSameDT=on
      settings: InputPortMap=u0,u1
  2-D Lookup Table2 : Lookup_n-D  BreakpointsForDimension1=atkinter  BreakpointsForDimension2=Minter  Table=caoff5000  InterpMethod=Cubic spline  ExtrapMethod=Clip  InternalRulePriority=Speed  RndMeth=Simplest  InputSameDT=on
      settings: InputPortMap=u0,u1
  2-D Lookup Table3 : Lookup_n-D  BreakpointsForDimension1=atkinter  BreakpointsForDimension2=Minter  Table=caon5000  InterpMethod=Cubic spline  ExtrapMethod=Clip  InternalRulePriority=Speed  RndMeth=Simplest  InputSameDT=on
      settings: InputPortMap=u0,u1
  2-D Lookup Table4 : Lookup_n-D  BreakpointsForDimension1=atkinter  BreakpointsForDimension2=Minter  Table=cl_phi5000  InterpMethod=Cubic spline  ExtrapMethod=Clip  InternalRulePriority=Speed  RndMeth=Simplest  InputSameDT=on
      settings: InputPortMap=u0,u1
  Mux : Mux  Inputs=10
  Output : Outport
  wires:
  1-D Lookup Table/1 -> Mux/5
  Mux/1 -> Output/1
  2-D Lookup Table2/1 -> Mux/2
  1-D Lookup Table2/1 -> Mux/6
  2-D Lookup Table/1 -> Mux/3
  2-D Lookup Table3/1 -> Mux/1
  2-D Lookup Table1/1 -> Mux/7
  1-D Lookup Table1/1 -> Mux/4
  Mach/1 -> 2-D Lookup Table3/2, 2-D Lookup Table2/2, 2-D Lookup Table/2, 1-D Lookup Table1/1, 1-D Lookup Table/1, 1-D Lookup Table2/1, 2-D Lookup Table4/2, 1-D Lookup Table4/1, 1-D Lookup Table3/1, 2-D Lookup Table1/2
  AOA/1 -> 2-D Lookup Table3/1, 2-D Lookup Table2/1, 2-D Lookup Table/1, 2-D Lookup Table4/1, 2-D Lookup Table1/1
  2-D Lookup Table4/1 -> Mux/10
  1-D Lookup Table4/1 -> Mux/9
  1-D Lookup Table3/1 -> Mux/8

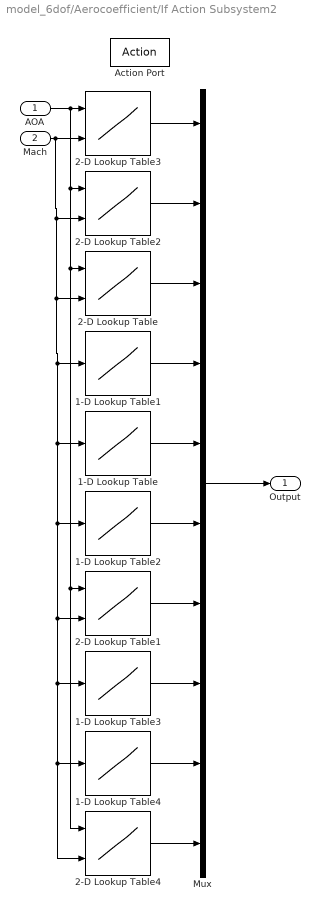
== system model_6dof/Aerocoefficient/If Action Subsystem2 ==
  AOA : Inport
  Mach : Inport  Port=2
  Action Port : ActionPort  ActionPortLabel=else
  1-D Lookup Table : Lookup_n-D  NumberOfTableDimensions=1  BreakpointsForDimension1=Minter  Table=cmq10000  InterpMethod=Cubic spline  ExtrapMethod=Clip  InternalRulePriority=Speed  RndMeth=Simplest  InputSameDT=on
  1-D Lookup Table1 : Lookup_n-D  NumberOfTableDimensions=1  BreakpointsForDimension1=Minter  Table=cnq10000  InterpMethod=Cubic spline  ExtrapMethod=Clip  InternalRulePriority=Speed  RndMeth=Simplest  InputSameDT=on
  1-D Lookup Table2 : Lookup_n-D  NumberOfTableDimensions=1  BreakpointsForDimension1=Minter  Table=cmdq10000  InterpMethod=Cubic spline  ExtrapMethod=Clip  InternalRulePriority=Speed  RndMeth=Simplest  InputSameDT=on
  1-D Lookup Table3 : Lookup_n-D  NumberOfTableDimensions=1  BreakpointsForDimension1=Minter  Table=cldp10000  InterpMethod=Cubic spline  ExtrapMethod=Clip  InternalRulePriority=Speed  RndMeth=Simplest  InputSameDT=on
  1-D Lookup Table4 : Lookup_n-D  NumberOfTableDimensions=1  BreakpointsForDimension1=Minter  Table=clp10000  InterpMethod=Cubic spline  ExtrapMethod=Clip  InternalRulePriority=Speed  RndMeth=Simplest  InputSameDT=on
  2-D Lookup Table : Lookup_n-D  BreakpointsForDimension1=atkinter  BreakpointsForDimension2=Minter  Table=cn10000  InterpMethod=Cubic spline  ExtrapMethod=Clip  InternalRulePriority=Speed  RndMeth=Simplest  InputSameDT=on
      settings: InputPortMap=u0,u1
  2-D Lookup Table1 : Lookup_n-D  BreakpointsForDimension1=atkinter  BreakpointsForDimension2=Minter  Table=Xcp10000  InterpMethod=Cubic spline  ExtrapMethod=Clip  InternalRulePriority=Speed  RndMeth=Simplest  InputSameDT=on
      settings: InputPortMap=u0,u1
  2-D Lookup Table2 : Lookup_n-D  BreakpointsForDimension1=atkinter  BreakpointsForDimension2=Minter  Table=caoff10000  InterpMethod=Cubic spline  ExtrapMethod=Clip  InternalRulePriority=Speed  RndMeth=Simplest  InputSameDT=on
      settings: InputPortMap=u0,u1
  2-D Lookup Table3 : Lookup_n-D  BreakpointsForDimension1=atkinter  BreakpointsForDimension2=Minter  Table=caon10000  InterpMethod=Cubic spline  ExtrapMethod=Clip  InternalRulePriority=Speed  RndMeth=Simplest  InputSameDT=on
      settings: InputPortMap=u0,u1
  2-D Lookup Table4 : Lookup_n-D  BreakpointsForDimension1=atkinter  BreakpointsForDimension2=Minter  Table=cl_phi10000  InterpMethod=Cubic spline  ExtrapMethod=Clip  InternalRulePriority=Speed  RndMeth=Simplest  InputSameDT=on
      settings: InputPortMap=u0,u1
  Mux : Mux  Inputs=10
  Output : Outport
  wires:
  1-D Lookup Table/1 -> Mux/5
  Mux/1 -> Output/1
  2-D Lookup Table2/1 -> Mux/2
  1-D Lookup Table2/1 -> Mux/6
  2-D Lookup Table/1 -> Mux/3
  2-D Lookup Table3/1 -> Mux/1
  2-D Lookup Table1/1 -> Mux/7
  1-D Lookup Table1/1 -> Mux/4
  Mach/1 -> 2-D Lookup Table4/2, 1-D Lookup Table4/1, 1-D Lookup Table3/1, 2-D Lookup Table1/2, 1-D Lookup Table2/1, 1-D Lookup Table/1, 1-D Lookup Table1/1, 2-D Lookup Table/2, 2-D Lookup Table2/2, 2-D Lookup Table3/2
  AOA/1 -> 2-D Lookup Table4/1, 2-D Lookup Table1/1, 2-D Lookup Table/1, 2-D Lookup Table2/1, 2-D Lookup Table3/1
  2-D Lookup Table4/1 -> Mux/10
  1-D Lookup Table4/1 -> Mux/9
  1-D Lookup Table3/1 -> Mux/8

== system model_6dof/EOM/quaternion kinetics ==
  wb : Inport
  Integrator4 : Integrator  InitialCondition=[e00;ex0;ey0;ez0]
  MATLAB Function3 : MATLAB Function  TreatAsAtomicUnit=on
  Normalization : dspmathops/Normalization  NormType=2-norm  Bias=1e-10  NormOver=Each column  Dimension=1  roundingMode=Floor  overflowMode=off  accumDataTypeStr=Inherit: Same as product output  accumLastDataTypeStr=Inherit: Same as product output  outputDataTypeStr=Inherit: Same as product output  outputMin=[]  outputMax=[]  outputLastDataTypeStr=Inherit: Same as product output
  Scope : Scope
  Scope1 : Scope
  Scope2 : Scope
  quat2angle : MATLAB Function  TreatAsAtomicUnit=on
  quat2angle1 : MATLAB Function  TreatAsAtomicUnit=on
  q : Outport
  angle : Outport  Port=2
  DCM_be : Outport  Port=3
  wires:
  wb/1 -> MATLAB Function3/1(wb)
  Integrator4/1 -> Scope2/1, Normalization/1
  Normalization/1 -> quat2angle1/1(q), quat2angle/1(q), MATLAB Function3/2(qb), q/1, Scope1/1
  MATLAB Function3/1(qbdot) -> Scope/1, Integrator4/1
  quat2angle/1(ang) -> angle/1
  quat2angle1/1(DCMbe) -> DCM_be/1

== system model_6dof/EOM/rotation dynamics ==
  I : Inport
  Mgt : Inport  Port=2
  ANG_ACC : Scope
  ANG_VEL : Scope
  Integrator3 : Integrator  InitialCondition=[p0;q0;r0]
  MATLAB Function2 : MATLAB Function  TreatAsAtomicUnit=on
  wb : Outport
  wires:
  Mgt/1 -> MATLAB Function2/3(Mgt)
  I/1 -> MATLAB Function2/1(I)
  Integrator3/1 -> MATLAB Function2/2(wb), ANG_VEL/1, wb/1
  MATLAB Function2/1(wbdot) -> ANG_ACC/1, Integrator3/1

== system model_6dof/EOM/transformation from body to NED ==
  vb : Inport
  q : Inport  Port=2
  Scope : Scope
  body to NED frame : MATLAB Function  TreatAsAtomicUnit=on
  ve : Outport
  wires:
  body to NED frame/1(ve) -> ve/1, Scope/1
  vb/1 -> body to NED frame/1(vb)
  q/1 -> body to NED frame/2(q)

== system model_6dof/EOM/translation dynamics ==
  m : Inport
  wb : Inport  Port=2
  Ft : Inport  Port=3
  ACC : Scope
  Integrator : Integrator  InitialCondition=[u0;v0;w0]
  Integrator5 : Integrator  InitialCondition=[x0;y0;z0]
  MATLAB Function1 : MATLAB Function  TreatAsAtomicUnit=on
  Scope3 : Scope
  VEL : Scope
  vb : Outport
  xb : Outport  Port=2
  ab : Outport  Port=3
  wires:
  wb/1 -> MATLAB Function1/3(wb)
  MATLAB Function1/1(vbdot) -> ACC/1, ab/1, Integrator/1
  Integrator/1 -> Integrator5/1, VEL/1, vb/1, MATLAB Function1/2(vb)
  Integrator5/1 -> Scope3/1, xb/1
  Ft/1 -> MATLAB Function1/4(Ft)
  m/1 -> MATLAB Function1/1(m)

== matlab function model_6dof/Enviroment/AOA calculate ==
  data: vb input; alpha output; beta output; alpha_t output; phi_w output; stage input
function [alpha, beta, alpha_t, phi_w] = fcn(vb, stage)
u = vb(1);
v = vb(2);
w = vb(3);

if(stage == 0) 
    alpha = 0;
    beta = 0;
    alpha_t = 0;
    phi_w = 0;
else
    alpha = atan2d(w,u);
    beta = atan2d(v,u);
    alpha_t = atan2d(sqrt(v^2+w^2),u);
    phi_w = atan2d(v,w);
end
end

== matlab function model_6dof/EOM/translation dynamics/MATLAB Function1 ==
  data: m input; vb input; vbdot output; wb input; Ft input
function vbdot = fcn(m,vb,wb,Ft)
p = wb(1);
q = wb(2);
r = wb(3);
CrossMat = [0   r   -q;
          -r    0    p;
           q  -p     0];
vbdot = Ft/m + CrossMat*vb;

== matlab function model_6dof/EOM/rotation dynamics/MATLAB Function2 ==
  data: I input; wbdot output; wb input; Mgt input
function wbdot = fcn(I,wb,Mgt)
p = wb(1);
q = wb(2);
r = wb(3);
Ixx = I(1);
Iyy = I(2);
Izz = I(3);
Imat = [Ixx    0    0;
          0  Iyy    0;
          0    0  Izz];
CrossMat = [0   r   -q;
          -r    0    p;
           q  -p     0];
wbdot = Imat\(Mgt + CrossMat*Imat*wb);

== matlab function model_6dof/EOM/quaternion kinetics/MATLAB Function3 ==
  data: wb input; qb input; qbdot output
function qbdot = fcn(wb,qb)
p = wb(1);
q = wb(2);
r = wb(3);
CrossMat = [0  -p  -q  -r;
            p   0   r  -q;
            q  -r   0   p;
            r   q  -p   0];
qbdot = 1/2*CrossMat*qb;

== matlab function model_6dof/EOM/transformation from body to NED/body to NED frame ==
  data: vb input; ve output; q input
function ve = fcn(vb,q)
e0 = q(1);
ex = q(2);
ey = q(3);
ez = q(4);
%% transform matrix for body frame to NED frame
Hbn = [e0^2+ex^2-ey^2-ez^2     2*(ex*ey-e0*ez)    2*(ex*ez+e0*ey);
       2*(ex*ey+e0*ez)     e0^2+ey^2-ex^2-ez^2    2*(ey*ez-e0*ex);
       2*(ex*ez-e0*ey)     2*(ey*ez+e0*ex)    e0^2+ez^2-ex^2-ey^2];
ve = Hbn*vb;

== matlab function model_6dof/Thrust command/thrust commend(0//1) ==
  data: thr input; t input; thr_cmd output
function thr_cmd = fcn(thr, t)
if t<5
    thr_cmd = 1;
else
    thr_cmd = 0;
end

== matlab function model_6dof/Actuator/MATLAB Function ==
  data: deltapyz input; delta1234 output; phi input
function delta1234 =  fcn(deltapyz,phi)

T = [-1  cosd(phi)-sind(phi) -sind(phi)-cosd(phi);
     -1  cosd(phi)+sind(phi) -sind(phi)+cosd(phi);
     -1 -cosd(phi)+sind(phi)  sind(phi)+cosd(phi);
     -1 -cosd(phi)-sind(phi)  sind(phi)-cosd(phi)];

delta1234 = T*deltapyz;

== matlab function model_6dof/EOM/quaternion kinetics/quat2angle ==
  data: q input; ang output
function ang = fcn(q)
q0 = q(1);
q1 = q(2);
q2 = q(3);
q3 = q(4);
phi = atan2(q2*q3+q0*q1,1/2-(q1^2+q2^2));
theta = asin(-2*(q1*q3-q0*q2));
psi = atan2(q1*q2+q0*q3,1/2-(q2^2+q3^2));
ang = [phi;theta;psi];

== matlab function model_6dof/EOM/quaternion kinetics/quat2angle1 ==
  data: q input; DCMbe output
function DCMbe = fcn(q)
e0 = q(1);
ex = q(2);
ey = q(3);
ez = q(4);
%% transform matrix for body frame to NED frame
Heb = [e0^2+ex^2-ey^2-ez^2     2*(ex*ey-e0*ez)    2*(ex*ez+e0*ey);
       2*(ex*ey+e0*ez)     e0^2+ey^2-ex^2-ez^2    2*(ey*ez-e0*ex);
       2*(ex*ez-e0*ey)     2*(ey*ez+e0*ex)    e0^2+ez^2-ex^2-ey^2];
DCMbe=Heb';

== matlab function model_6dof/F&M/MATLAB Function ==
  data: moment input; fac output; XCG input; Xcpcanard input; qbar input; l output
function [fac,l] = fcn(moment,XCG,Xcpcanard,qbar)
l = Xcpcanard*0.265 - XCG;
fac = moment/(qbar*l);
